simulink model "Motor_regeneative_different_load"  (R2016a)
settings: Solver=VariableStepAuto  StartTime=0.0  StopTime=120  FixedStep=2  RelTol=1e-3
libraries: simulink x1
settings Model: Creator=Dell  LastModifiedBy=Dell

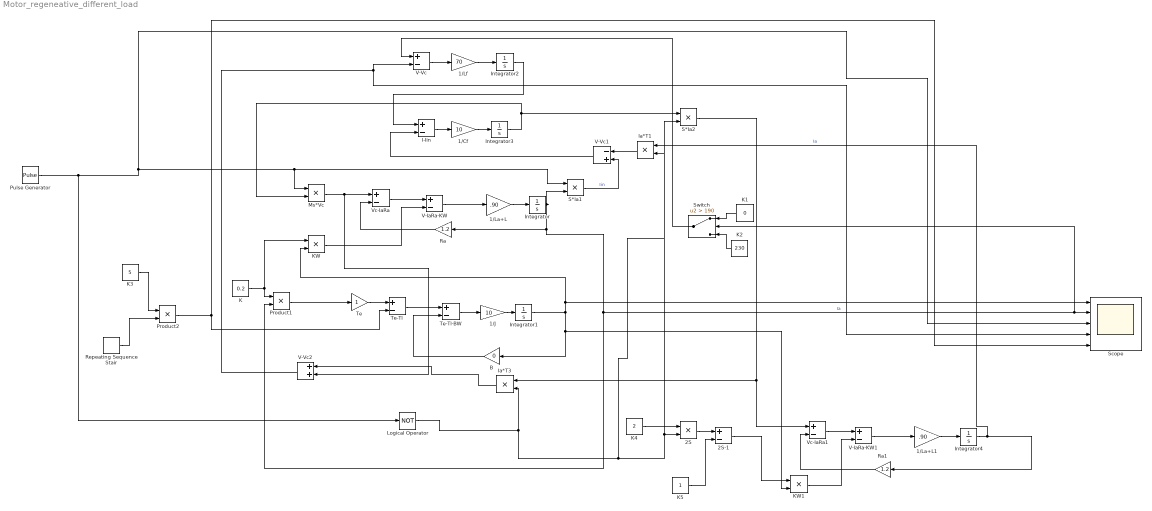
== system Motor_regeneative_different_load ==
  1/Cf : Gain  Gain=10
  1/J : Gain  Gain=10
  1/La+L : Gain  Gain=.90
  1/La+L1 : Gain  Gain=.90
  1/Lf : Gain  Gain=70
  2S : Product
  2S-1 : Sum  Inputs=+-
  B : Gain  Gain=0
  I-Iin : Sum  Inputs=+-
  Ia*T1 : Product
  Ia*T3 : Product
  Integrator{,1..4} (5 alike) : Integrator
  K : Constant  Value=0.2
  K1 : Constant  Value=0
  K2 : Constant  Value=230
  K3 : Constant  Value=5
  K4 : Constant  Value=2
  K5 : Constant
  KW : Product
  KW1 : Product
  Logical Operator : Logic  Operator=NOT  AllPortsSameDT=off  OutDataTypeStr=boolean
  Ms*Vc : Product
  Product1 : Product
  Product2 : Product
  Pulse Generator : DiscretePulseGenerator  PulseType=Time based  Period=80  PulseWidth=98
  Ra : Gain  Gain=1.2
  Ra1 : Gain  Gain=1.2
  Repeating Sequence Stair : simulink/Sources/Repeating Sequence Stair  OutValues=[0 1 4 2 1].'  tsamp=30  OutMin=[]  OutMax=[]  OutDataTypeStr=double  OutputDataTypeScalingMode=double  OutDataType=fixdt(0,8)  ConRadixGroup=Best Precision: Vector-wise  OutScaling=2^-12
  S*Ia1 : Product
  S*Ia2 : Product
  Scope : Scope  NumInputPorts=5
  Switch : Switch  Criteria=u2 > Threshold  Threshold=190
  Te : Gain
  Te-Tl : Sum  Inputs=+-
  Te-Tl-BW : Sum  Inputs=+-
  V-IaRa-KW : Sum  Inputs=+-
  V-IaRa-KW1 : Sum  Inputs=+-
  V-Vc : Sum  Inputs=+-
  V-Vc1 : Sum  Inputs=-+
  V-Vc2 : Sum
  Vc-IaRa : Sum  Inputs=+-
  Vc-IaRa1 : Sum  Inputs=+-
  wires:
  Integrator2/1 -> I-Iin/1
  V-Vc/1 -> 1/Lf/1
  1/Lf/1 -> Integrator2/1
  1/Cf/1 -> Integrator3/1
  KW/1 -> V-IaRa-KW/2
  1/La+L/1 -> Integrator/1
  B/1 -> Te-Tl-BW/2
  Ra/1 -> Vc-IaRa/2
  V-IaRa-KW/1 -> 1/La+L/1
  Vc-IaRa/1 -> V-IaRa-KW/1
  Te-Tl/1 -> Te-Tl-BW/1
  Product1/1 -> Te/1
  K/1 -> KW/1, Product1/1
  Te-Tl-BW/1 -> 1/J/1
  Integrator/1 -> S*Ia1/2, Product1/2, Switch/2, Scope/2, Ra/1  "Ia"
  Te/1 -> Te-Tl/1
  1/J/1 -> Integrator1/1
  Integrator1/1 -> KW/2, Scope/1, KW1/2, B/1
  KW1/1 -> V-IaRa-KW1/2
  1/La+L1/1 -> Integrator4/1
  Ra1/1 -> Vc-IaRa1/2
  V-IaRa-KW1/1 -> 1/La+L1/1
  Vc-IaRa1/1 -> V-IaRa-KW1/1
  Integrator4/1 -> Ra1/1, Ia*T1/1  "Ia"
  K4/1 -> 2S/1
  2S/1 -> 2S-1/1
  K5/1 -> 2S-1/2
  Integrator3/1 -> S*Ia2/1, Ms*Vc/2
  Pulse Generator/1 -> Scope/3, Ms*Vc/1, S*Ia1/1, Logical Operator/1
  I-Iin/1 -> 1/Cf/1
  2S-1/1 -> KW1/1
  Logical Operator/1 -> 2S/2, S*Ia2/2, Ia*T1/2, Ia*T3/2
  V-Vc1/1 -> I-Iin/2
  S*Ia2/1 -> Ia*T3/1, Vc-IaRa1/1
  Ms*Vc/1 -> V-Vc2/2, Vc-IaRa/1
  Ia*T3/1 -> V-Vc2/1
  V-Vc2/1 -> Scope/4, V-Vc/2
  Product2/1 -> Te-Tl/2, Scope/5
  Ia*T1/1 -> V-Vc1/1
  S*Ia1/1 -> V-Vc1/2  "Iin"
  K2/1 -> Switch/3
  K1/1 -> Switch/1
  Switch/1 -> V-Vc/1
  K3/1 -> Product2/1
  Repeating Sequence Stair/1 -> Product2/2
